simulink model "nonlinear"  (R2024b)
settings: Solver=FixedStepAuto  StartTime=0.0  StopTime=250  FixedStep=0.01  RelTol=1e-3
settings Model: Creator=castl  LastModifiedBy=castl

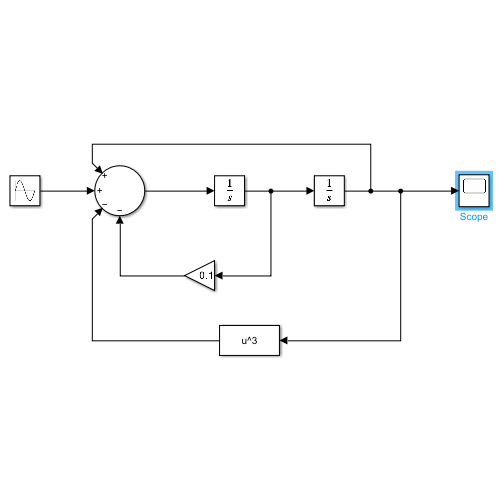
[thumbnail: Simulink's stored preview of the top-level diagram]
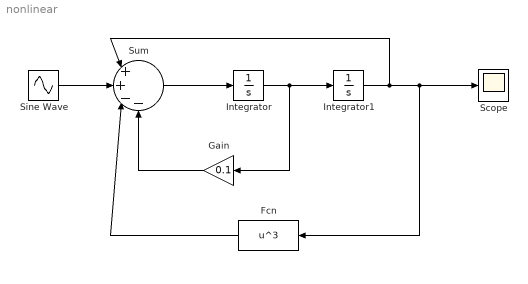
== system nonlinear ==
  Fcn : Fcn  Expr=u^3
  Gain : Gain  Gain=0.1
  Integrator : Integrator  InitialCondition=0.29
  Integrator1 : Integrator  InitialCondition=0.585
  Scope : Scope
  Sine Wave : Sin  Amplitude=0.07  Frequency=1.25  Phase=pi/2  SampleTime=0
  Sum : Sum  Inputs=|++--
  wires:
  Sine Wave/1 -> Sum/2
  Sum/1 -> Integrator/1
  Integrator/1 -> Gain/1, Integrator1/1
  Gain/1 -> Sum/4
  Integrator1/1 -> Sum/1, Fcn/1, Scope/1
  Fcn/1 -> Sum/3
